simulink library "MEKF_ValidityTest_Lib2018"  (R2018b)
settings: Solver=VariableStepAuto  StartTime=0.0  StopTime=10.0  RelTol=1e-3
values from neighbouring files (symbols this model uses):
  Beta_init = Beta    [MEKF_ScriptandSimulink_Test.m]
  del_t = tspan(2)-tspan(1)    [MEKF_ScriptandSimulink_Test.m]
  P_sq_init = P_sq    [MEKF_ScriptandSimulink_Test.m]
  q = [q(:,2),q(:,3),q(:,4),q(:,1)]    [MEKF_ScriptandSimulink_Test.m]
  Q_sq = chol((gamma*Q_k*gamma'),'lower')    [MEKF_ScriptandSimulink_Test.m]
  qe_init = qe    [MEKF_ScriptandSimulink_Test.m]
  R_sq = chol(R,'lower')    [MEKF_ScriptandSimulink_Test.m]
libraries: MEKF_LibraryR2018b x13, aerolibutil x12, dspmtrx3 x7, sharedutil x6, $bdroot x2
(part 1 of 2)
settings Model: Creator=kylle  LastModifiedBy=kylle
settings DataIOCC: ReturnWorkspaceOutputs=on

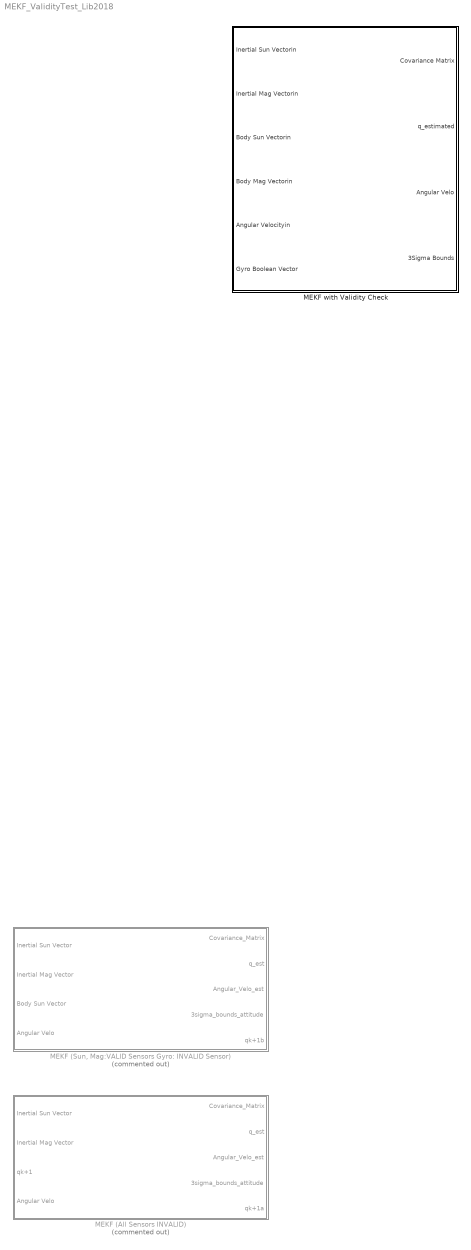
== system MEKF_ValidityTest_Lib2018 ==
  MEKF (All Sensors INVALID) : Subsystem  Commented=on  AncestorBlock=MEKF_Propagation_Lib/MEKF (Gyro Sensors Work, Mag or Sun sensors INVALID)
  "MEKF (Sun, Mag:VALID Sensors Gyro: INVALID Sensor)" : Subsystem  Commented=on  AncestorBlock=MEKF_Propagation_Lib/Multiplicative Extended Kalman Filter (all Valid Sensors)
  MEKF with Validity Check : Subsystem

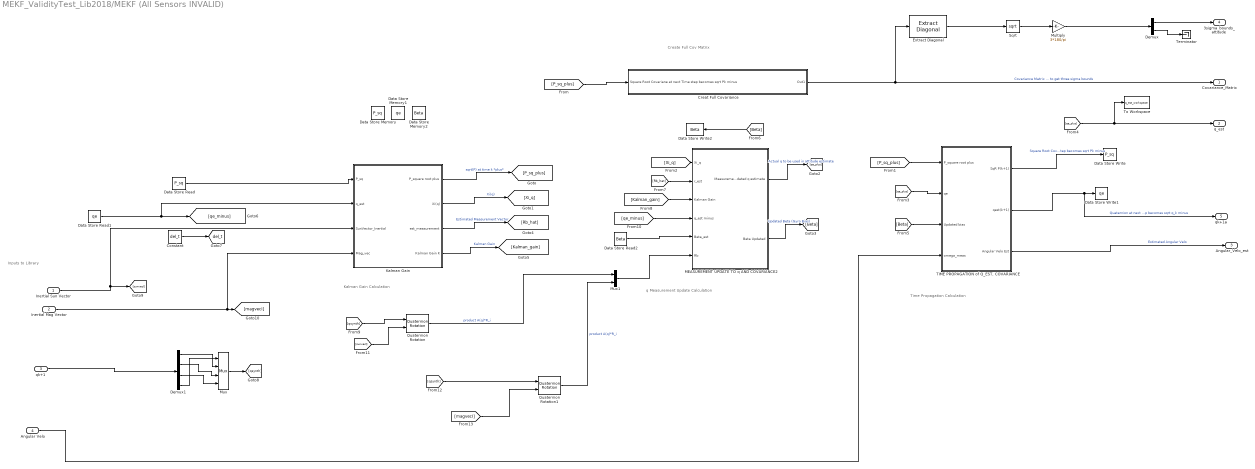
== system MEKF_ValidityTest_Lib2018/MEKF (All Sensors INVALID) ==
  note: Create Full Cov Matrix
  note: Time Propagation Calculation
  note: q Measurement Update Calculation
  note: Inputs to Library
  note: Kalman Gain Calculation
  Inertial Sun Vector : Inport
  Inertial Mag Vector : Inport  Port=2
  qk+1 : Inport  Port=3
  Angular Velo : Inport  Port=4
  Constant : Constant  Value=del_t
  Creat Full Covariance : Subsystem
  Data Store Memory : DataStoreMemory  DataStoreName=P_sq  InitialValue=P_sq_init  VectorParams1D=off  ShowAdditionalParam=off
  Data Store Memory1 : DataStoreMemory  DataStoreName=qe  InitialValue=1000  VectorParams1D=off  ShowAdditionalParam=off
  Data Store Memory2 : DataStoreMemory  DataStoreName=Beta  InitialValue=Beta_init  VectorParams1D=off  ShowAdditionalParam=off
  Data Store Read : DataStoreRead  DataStoreName=P_sq
  Data Store Read1 : DataStoreRead  DataStoreName=qe
  Data Store Read2 : DataStoreRead  DataStoreName=Beta
  Data Store Write : DataStoreWrite  DataStoreName=P_sq
  Data Store Write1 : DataStoreWrite  DataStoreName=qe
  Data Store Write2 : DataStoreWrite  DataStoreName=Beta
  Demux : Demux  Outputs=2
  Demux1 : Demux
  Extract Diagonal : dspmtrx3/Extract Diagonal
      settings: SourceProductName=DSP System Toolbox  SourceProductBaseCode=DS
  Kalman Gain : Subsystem
  MEASUREMENT UPDATE TO q AND COVARIANCE2 : Subsystem
  Multiply : Gain  Gain=3*180/pi
  Mux : Mux
  Mux1 : Mux  Inputs=2
  Quaternion Rotation : aerolibutil/Quaternion Rotation
  Quaternion Rotation1 : aerolibutil/Quaternion Rotation
  Sqrt : Sqrt  SaturateOnIntegerOverflow=on
  "TIME PROPAGATION of Q_EST, COVARIANCE" : Subsystem
  Terminator : Terminator
  To Workspace : ToWorkspace  VariableName=q_est_workspace  SaveFormat=Timeseries  SampleTime=-1
  Covariance_Matrix : Outport
  q_est : Outport  Port=2
  Angular_Velo_est : Outport  Port=3
  3sigma_bounds_attitude : Outport  Port=4
  qk+1a : Outport  Port=5
  tag scope: del_t=global
  wires:
  Data Store Read1/1 -> [qe_minus], Kalman Gain/2(q_est)
  Inertial Mag Vector/1 -> [magvecI], Kalman Gain/4("Mag_vec ")
  Demux/2 -> Terminator/1
  Demux/1 -> 3sigma_bounds_attitude/1
  Multiply/1 -> Demux/1
  Sqrt/1 -> Multiply/1
  Extract Diagonal/1 -> Sqrt/1
  Creat Full Covariance/1(Out1) -> Covariance_Matrix/1, Extract Diagonal/1  "Covariance Matrix from which to get three sigma bounds"
  "TIME PROPAGATION of Q_EST, COVARIANCE"/3(Angular Velo Est) -> Angular_Velo_est/1  "Estimated Angular Velo"
  Angular Velo/1 -> "TIME PROPAGATION of Q_EST, COVARIANCE"/4(omega_meas)
  Kalman Gain/4(Kalman Gain K) -> [Kalman_gain]  "Kalman Gain"
  Inertial Sun Vector/1 -> [sunvecI], Kalman Gain/3(SunVector_Inertial)
  MEASUREMENT UPDATE TO q AND COVARIANCE2/2(Beta Updated) -> [Beta]  "Updated Beta (Gyro Bias)"
  Kalman Gain/3(est_measurement) -> [Rb_hat]  "Estimated Measurement Vector"
  Data Store Read2/1 -> MEASUREMENT UPDATE TO q AND COVARIANCE2/5(Beta_est)
  MEASUREMENT UPDATE TO q AND COVARIANCE2/1(Measurement updated q estimate) -> [qe_plus]  "Actual q to be used in attitude estimate"
  Kalman Gain/1(P_square root plus) -> [P_sq_plus]  "sqrt(P) at time k *plus*"
  [Kalman_gain] -> MEASUREMENT UPDATE TO q AND COVARIANCE2/3(Kalman Gain)
  [qe_minus] -> MEASUREMENT UPDATE TO q AND COVARIANCE2/4(q_est minus)
  [qe_plus] -> "TIME PROPAGATION of Q_EST, COVARIANCE"/2(qe)
  [P_sq_plus] -> "TIME PROPAGATION of Q_EST, COVARIANCE"/1(P_square root plus)
  [Xi_q] -> MEASUREMENT UPDATE TO q AND COVARIANCE2/1(Xi_q)
  Constant/1 -> [del_t]
  "TIME PROPAGATION of Q_EST, COVARIANCE"/1(SqR P(k+1)) -> Data Store Write/1  "Square Root Covariane at next Time step becomes sqrt Pk minus"
  [P_sq_plus] -> Creat Full Covariance/1(Square Root Covariane at next Time step becomes sqrt Pk minus)
  [Beta] -> "TIME PROPAGATION of Q_EST, COVARIANCE"/3(Updated bias)
  [Beta] -> Data Store Write2/1
  Kalman Gain/2(Xi(q)) -> [Xi_q]  "Xi(q)"
  "TIME PROPAGATION of Q_EST, COVARIANCE"/2(qest(k+1)) -> qk+1a/1, Data Store Write1/1  "Quaternion at next Time step becomes sqrt q_k minus"
  Data Store Read/1 -> Kalman Gain/1(P_sq)
  [Rb_hat] -> MEASUREMENT UPDATE TO q AND COVARIANCE2/2(r_est)
  [qe_plus] -> To Workspace/1, q_est/1
  qk+1/1 -> Demux1/1
  Quaternion Rotation/1 -> Mux1/1  "product A(q)*R_i"
  [sunvecI] -> Quaternion Rotation/2
  Demux1/2 -> Mux/3
  Mux/1 -> [qsynth]
  Demux1/3 -> Mux/4
  Demux1/1 -> Mux/2
  Demux1/4 -> Mux/1
  [qsynth] -> Quaternion Rotation/1
  Quaternion Rotation1/1 -> Mux1/2  "product A(q)*R_i"
  [qsynth] -> Quaternion Rotation1/1
  [magvecI] -> Quaternion Rotation1/2
  Mux1/1 -> MEASUREMENT UPDATE TO q AND COVARIANCE2/6(Rb)

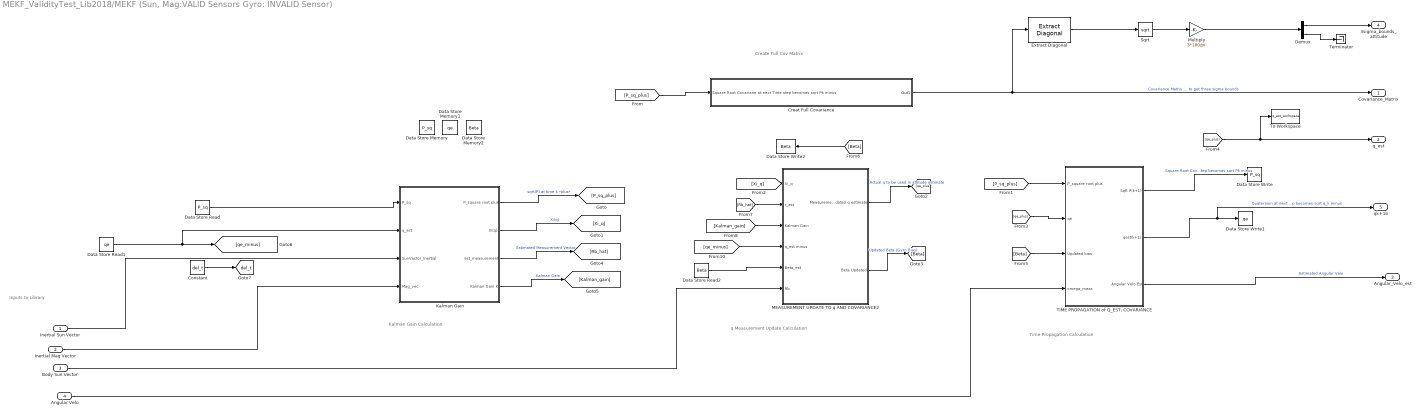
== system MEKF_ValidityTest_Lib2018/MEKF (Sun, Mag:VALID Sensors Gyro: INVALID Sensor) ==
  note: Kalman Gain Calculation
  note: Inputs to Library
  note: q Measurement Update Calculation
  note: Time Propagation Calculation
  note: Create Full Cov Matrix
  Inertial Sun Vector : Inport
  Inertial Mag Vector : Inport  Port=2
  Body Sun Vector : Inport  Port=3
  Angular Velo : Inport  Port=4
  Constant : Constant  Value=del_t
  Creat Full Covariance : Subsystem
  Data Store Memory : DataStoreMemory  DataStoreName=P_sq  InitialValue=P_sq_init  VectorParams1D=off  ShowAdditionalParam=off
  Data Store Memory1 : DataStoreMemory  DataStoreName=qe  InitialValue=1000  VectorParams1D=off  ShowAdditionalParam=off
  Data Store Memory2 : DataStoreMemory  DataStoreName=Beta  InitialValue=Beta_init  VectorParams1D=off  ShowAdditionalParam=off
  Data Store Read : DataStoreRead  DataStoreName=P_sq
  Data Store Read1 : DataStoreRead  DataStoreName=qe
  Data Store Read2 : DataStoreRead  DataStoreName=Beta
  Data Store Write : DataStoreWrite  DataStoreName=P_sq
  Data Store Write1 : DataStoreWrite  DataStoreName=qe
  Data Store Write2 : DataStoreWrite  DataStoreName=Beta
  Demux : Demux  Outputs=2
  Extract Diagonal : dspmtrx3/Extract Diagonal
      settings: SourceProductName=DSP System Toolbox  SourceProductBaseCode=DS
  Kalman Gain : Subsystem
  MEASUREMENT UPDATE TO q AND COVARIANCE2 : Subsystem
  Multiply : Gain  Gain=3*180/pi
  Sqrt : Sqrt  SaturateOnIntegerOverflow=on
  "TIME PROPAGATION of Q_EST, COVARIANCE" : Subsystem
  Terminator : Terminator
  To Workspace : ToWorkspace  VariableName=q_est_workspace  SaveFormat=Timeseries  SampleTime=-1
  Covariance_Matrix : Outport
  q_est : Outport  Port=2
  Angular_Velo_est : Outport  Port=3
  3sigma_bounds_attitude : Outport  Port=4
  qk+1b : Outport  Port=5
  tag scope: del_t=global
  wires:
  [qe_plus] -> q_est/1, To Workspace/1
  [Rb_hat] -> MEASUREMENT UPDATE TO q AND COVARIANCE2/2(r_est)
  Data Store Read/1 -> Kalman Gain/1(P_sq)
  "TIME PROPAGATION of Q_EST, COVARIANCE"/2(qest(k+1)) -> qk+1b/1, Data Store Write1/1  "Quaternion at next Time step becomes sqrt q_k minus"
  Kalman Gain/2(Xi(q)) -> [Xi_q]  "Xi(q)"
  [Beta] -> Data Store Write2/1
  [Beta] -> "TIME PROPAGATION of Q_EST, COVARIANCE"/3(Updated bias)
  [P_sq_plus] -> Creat Full Covariance/1(Square Root Covariane at next Time step becomes sqrt Pk minus)
  "TIME PROPAGATION of Q_EST, COVARIANCE"/1(SqR P(k+1)) -> Data Store Write/1  "Square Root Covariane at next Time step becomes sqrt Pk minus"
  Constant/1 -> [del_t]
  [Xi_q] -> MEASUREMENT UPDATE TO q AND COVARIANCE2/1(Xi_q)
  [P_sq_plus] -> "TIME PROPAGATION of Q_EST, COVARIANCE"/1(P_square root plus)
  [qe_plus] -> "TIME PROPAGATION of Q_EST, COVARIANCE"/2(qe)
  [qe_minus] -> MEASUREMENT UPDATE TO q AND COVARIANCE2/4(q_est minus)
  [Kalman_gain] -> MEASUREMENT UPDATE TO q AND COVARIANCE2/3(Kalman Gain)
  Kalman Gain/1(P_square root plus) -> [P_sq_plus]  "sqrt(P) at time k *plus*"
  MEASUREMENT UPDATE TO q AND COVARIANCE2/1(Measurement updated q estimate) -> [qe_plus]  "Actual q to be used in attitude estimate"
  Data Store Read2/1 -> MEASUREMENT UPDATE TO q AND COVARIANCE2/5(Beta_est)
  Kalman Gain/3(est_measurement) -> [Rb_hat]  "Estimated Measurement Vector"
  MEASUREMENT UPDATE TO q AND COVARIANCE2/2(Beta Updated) -> [Beta]  "Updated Beta (Gyro Bias)"
  Inertial Sun Vector/1 -> Kalman Gain/3(SunVector_Inertial)
  Kalman Gain/4(Kalman Gain K) -> [Kalman_gain]  "Kalman Gain"
  Angular Velo/1 -> "TIME PROPAGATION of Q_EST, COVARIANCE"/4(omega_meas)
  "TIME PROPAGATION of Q_EST, COVARIANCE"/3(Angular Velo Est) -> Angular_Velo_est/1  "Estimated Angular Velo"
  Creat Full Covariance/1(Out1) -> Extract Diagonal/1, Covariance_Matrix/1  "Covariance Matrix from which to get three sigma bounds"
  Extract Diagonal/1 -> Sqrt/1
  Sqrt/1 -> Multiply/1
  Multiply/1 -> Demux/1
  Demux/1 -> 3sigma_bounds_attitude/1
  Demux/2 -> Terminator/1
  Body Sun Vector/1 -> MEASUREMENT UPDATE TO q AND COVARIANCE2/6(Rb)
  Inertial Mag Vector/1 -> Kalman Gain/4("Mag_vec ")
  Data Store Read1/1 -> Kalman Gain/2(q_est), [qe_minus]

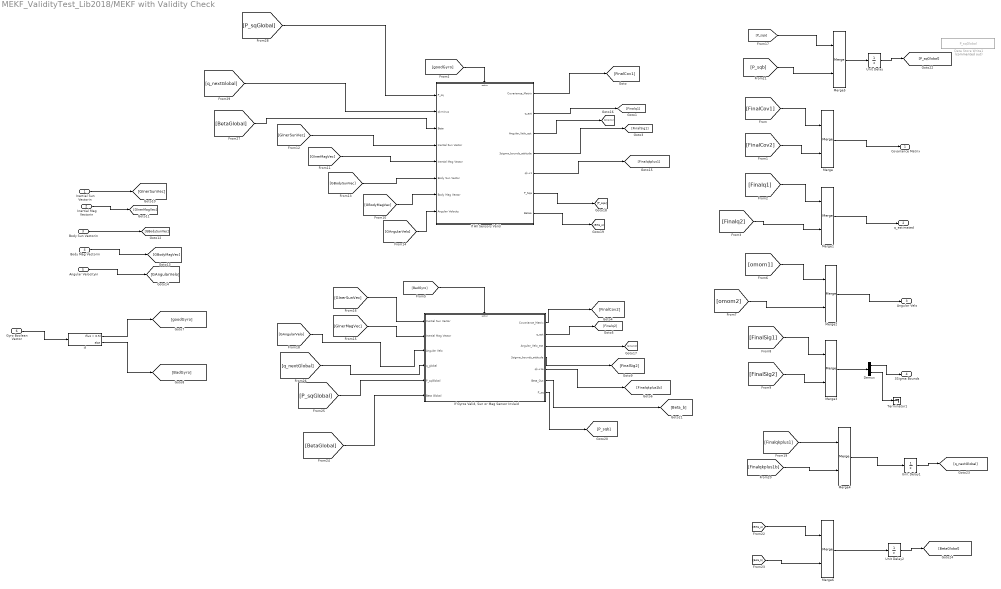
== system MEKF_ValidityTest_Lib2018/MEKF with Validity Check ==
  Inertial Sun Vectorin : Inport
  Inertial Mag Vectorin : Inport  Port=2
  Body Sun Vectorin : Inport  Port=3
  Body Mag Vectorin : Inport  Port=4
  Angular Velocityin : Inport  Port=5
  Gyro Boolean Vector : Inport  Port=6
  Data Store Write1 : DataStoreWrite  Commented=on  DataStoreName=P_sqGlobal
  Demux : Demux  Outputs=2
  If : If  IfExpression=u1 > 0.5
  If All Sensors Valid : Subsystem  TreatAsAtomicUnit=on
  "If Gyros Valid, Sun or Mag Sensor Invlaid" : Subsystem  TreatAsAtomicUnit=on
  Merge{,1..6} (7 alike) : Merge
  Terminator1 : Terminator
  Unit Delay : UnitDelay  InitialCondition=P_sq_init  SampleTime=-1  HasFrameUpgradeWarning=on
  Unit Delay1 : UnitDelay  InitialCondition=qe_init  SampleTime=-1  HasFrameUpgradeWarning=on
  Unit Delay2 : UnitDelay  InitialCondition=Beta_init  SampleTime=-1  HasFrameUpgradeWarning=on
  Covariance Matrix : Outport
  q_estimated : Outport  Port=2
  Angular Velo : Outport  Port=3
  3Sigma Bounds : Outport  Port=4
  wires:
  [GBodySunVec] -> If All Sensors Valid/6(Body Sun Vector)
  [FinalCov2] -> Merge/2
  [GInerMagVec] -> "If Gyros Valid, Sun or Mag Sensor Invlaid"/2(Inertial Mag Vector)
  Gyro Boolean Vector/1 -> If/1
  [GInerMagVec] -> If All Sensors Valid/5(Inertial Mag Vector)
  Body Mag Vectorin/1 -> [GBodyMagVec]
  Merge1/1 -> q_estimated/1
  [GBodyMagVec] -> If All Sensors Valid/7(Body Mag Vector)
  [FinalSig2] -> Merge3/2
  Body Sun Vectorin/1 -> [GBodySunVec]
  [GAngularVelo] -> If All Sensors Valid/8(Angular Velocity)
  "If Gyros Valid, Sun or Mag Sensor Invlaid"/5(qk+1a) -> [Finalqkplus1b]
  If All Sensors Valid/2(q_est) -> [Finalq1]
  If All Sensors Valid/1(Covariance_Matrix) -> [FinalCov1]
  [FinalSig1] -> Merge3/1
  Angular Velocityin/1 -> [GAngularVelo]
  [BadGyro] -> "If Gyros Valid, Sun or Mag Sensor Invlaid"/Action
  [GInerSunVec] -> "If Gyros Valid, Sun or Mag Sensor Invlaid"/1(Inertial Sun Vector)
  [GAngularVelo] -> "If Gyros Valid, Sun or Mag Sensor Invlaid"/3(Angular Velo)
  If All Sensors Valid/4(3sigma_bounds_attitude) -> [FinalSig1]
  Inertial Sun Vectorin/1 -> [GInerSunVec]
  "If Gyros Valid, Sun or Mag Sensor Invlaid"/2(q_est) -> [Finalq2]
  [GInerSunVec] -> If All Sensors Valid/4(Inertial Sun Vector)
  Merge2/1 -> Angular Velo/1
  "If Gyros Valid, Sun or Mag Sensor Invlaid"/1(Covariance_Matrix) -> [FinalCov2]
  [goodGyro] -> If All Sensors Valid/Action
  [Finalq1] -> Merge1/1
  "If Gyros Valid, Sun or Mag Sensor Invlaid"/4(3sigma_bounds_attitude) -> [FinalSig2]
  Merge/1 -> Covariance Matrix/1
  [FinalCov1] -> Merge/1
  [q_nextGlobal] -> "If Gyros Valid, Sun or Mag Sensor Invlaid"/4(q_global)
  Inertial Mag Vectorin/1 -> [GInerMagVec]
  If All Sensors Valid/5(qk+1) -> [Finalqkplus1]
  Merge3/1 -> Demux/1
  Demux/1 -> 3Sigma Bounds/1
  Demux/2 -> Terminator1/1
  [P_sqGlobal] -> "If Gyros Valid, Sun or Mag Sensor Invlaid"/5(P_sqGlobal)
  [Finalqkplus1] -> Merge4/1
  [Finalqkplus1b] -> Merge4/2
  [BetaGlobal] -> "If Gyros Valid, Sun or Mag Sensor Invlaid"/6(Beta Global)
  [BetaGlobal] -> If All Sensors Valid/3(Beta)
  [omom1] -> Merge2/1
  If All Sensors Valid/3(Angular_Velo_est) -> [omom1]
  If All Sensors Valid/6("P_Sqa ") -> [P_sqa]
  If All Sensors Valid/7(Betaa) -> [Beta_a]
  [P_sqa] -> Merge5/1
  "If Gyros Valid, Sun or Mag Sensor Invlaid"/7(P_sq) -> [P_sqb]
  "If Gyros Valid, Sun or Mag Sensor Invlaid"/6(Beta_Out) -> [Beta_b]
  [P_sqb] -> Merge5/2
  "If Gyros Valid, Sun or Mag Sensor Invlaid"/3(Angular_Velo_est) -> [omom2]
  [omom2] -> Merge2/2
  [Beta_a] -> Merge6/1
  [Beta_b] -> Merge6/2
  Merge5/1 -> Unit Delay/1
  Unit Delay/1 -> [P_sqGlobal]
  Unit Delay1/1 -> [q_nextGlobal]
  Merge4/1 -> Unit Delay1/1
  Unit Delay2/1 -> [BetaGlobal]
  Merge6/1 -> Unit Delay2/1
  [q_nextGlobal] -> If All Sensors Valid/2(qkminus)
  [P_sqGlobal] -> If All Sensors Valid/1(P_sq)
  If/1 -> [goodGyro]
  If/2 -> [BadGyro]
  [Finalq2] -> Merge1/2

== system MEKF_ValidityTest_Lib2018/MEKF (All Sensors INVALID)/Creat Full Covariance ==
  Square Root Covariane at next Time step becomes sqrt Pk minus : Inport
  Matrix Multiply : Product  Multiplication=Matrix(*)
  Transpose : Math  Operator=transpose  SaturateOnIntegerOverflow=on
  Out1 : Outport
  wires:
  Matrix Multiply/1 -> Out1/1
  Transpose/1 -> Matrix Multiply/2
  Square Root Covariane at next Time step becomes sqrt Pk minus/1 -> Matrix Multiply/1, Transpose/1

== system MEKF_ValidityTest_Lib2018/MEKF (All Sensors INVALID)/Kalman Gain ==
  P_sq : Inport
  q_est : Inport  Port=2
  SunVector_Inertial : Inport  Port=3
  "Mag_vec " : Inport  Port=4
  Constant : Constant  Value=R_sq*10000  VectorParams1D=off
  Create H matrix : Subsystem
  Demux : Demux
  Divide : Product  Inputs=/  Multiplication=Matrix(*)
  MATLAB Function2 : MATLAB Function  TreatAsAtomicUnit=on
  MATLAB Function3 : MATLAB Function  Commented=on  TreatAsAtomicUnit=on
  MATLAB Function4 : MATLAB Function  Commented=on  TreatAsAtomicUnit=on
  Makes Xi(q) Matrix : Subsystem
  Matrix Concatenate : Concatenate  Mode=Multidimensional array
  Matrix Multiply1 : Product  Multiplication=Matrix(*)
  Mux : Mux
  Quaternion Rotation : aerolibutil/Quaternion Rotation
  Quaternion Rotation1 : aerolibutil/Quaternion Rotation
  P_square root plus : Outport
  Xi(q) : Outport  Port=2
  est_measurement : Outport  Port=3
  Kalman Gain K : Outport  Port=4
  wires:
  Matrix Concatenate/1 -> est_measurement/1
  [bhat] -> Matrix Concatenate/2
  [rb_hat] -> Matrix Concatenate/1
  [bhat] -> Create H matrix/2(bb_hat)
  [qmix] -> Quaternion Rotation/1
  [qmix] -> Quaternion Rotation1/1
  Mux/1 -> [qmix]
  Quaternion Rotation1/1 -> [bhat]  "product A(q)*B_i"
  "Mag_vec "/1 -> Quaternion Rotation1/2
  [rb_hat] -> Create H matrix/1(rb_hat)
  Quaternion Rotation/1 -> [rb_hat]  "product A(q)*R_i"
  [q_est] -> Makes Xi(q) Matrix/1(qest)
  [q_est] -> Demux/1
  q_est/1 -> [q_est]
  Makes Xi(q) Matrix/1(Xi(q)) -> Xi(q)/1
  Demux/4 -> Mux/1
  Demux/3 -> Mux/4
  Demux/2 -> Mux/3
  Demux/1 -> Mux/2
  MATLAB Function2/3(P_sq) -> P_square root plus/1  "P_square root plus"
  Constant/1 -> MATLAB Function2/1(R_sq)
  SunVector_Inertial/1 -> Quaternion Rotation/2
  Matrix Multiply1/1 -> Kalman Gain K/1  "Kalman Gain K"
  P_sq/1 -> MATLAB Function2/2("P_sq ")
  MATLAB Function2/2(sq_Bk) -> Divide/1
  Create H matrix/1(H) -> MATLAB Function2/3(H)  "Sensitivity Matrix"
  MATLAB Function2/1(W) -> Matrix Multiply1/1
  Divide/1 -> Matrix Multiply1/2

== system MEKF_ValidityTest_Lib2018/MEKF (All Sensors INVALID)/MEASUREMENT UPDATE TO q AND COVARIANCE2 ==
  Xi_q : Inport
  r_est : Inport  Port=2
  Kalman Gain : Inport  Port=3
  q_est minus : Inport  Port=4
  Beta_est : Inport  Port=5
  Rb : Inport  Port=6
  Create Measurement Residual : Sum  Inputs=+-
  Demux : Demux  Outputs=2
  Normalize_q : Subsystem
  Product : Product  Inputs=**  Multiplication=Matrix(*)
  Product1 : Product  Multiplication=Matrix(*)
  Sum : Sum  Inputs=|++
  "Updating Beta Bias " : Sum  Inputs=|++
  gain1 : Gain  Gain=0.5
  Measurement updated q estimate : Outport
  Beta Updated : Outport  Port=2
  wires:
  Normalize_q/1(q_normalized) -> Measurement updated q estimate/1
  Sum/1 -> Normalize_q/1(Estimated Quaternion)  "Estimated Quaternion"
  Xi_q/1 -> gain1/1  "quaternion Propagation Matrix"
  Rb/1 -> Create Measurement Residual/1
  Kalman Gain/1 -> Product1/1
  q_est minus/1 -> Sum/2
  Beta_est/1 -> "Updating Beta Bias "/2  "Beta_estimated"
  "Updating Beta Bias "/1 -> Beta Updated/1  "Beta Updated"
  Create Measurement Residual/1 -> Product1/2  "Measurement Residual"
  r_est/1 -> Create Measurement Residual/2
  Product1/1 -> Demux/1  "del_x"
  Product/1 -> Sum/1
  Demux/2 -> "Updating Beta Bias "/1  "Delta Beta"
  gain1/1 -> Product/1  "0.5*Xi_q"
  Demux/1 -> Product/2  "Delta Alpha"

== system MEKF_ValidityTest_Lib2018/MEKF (All Sensors INVALID)/TIME PROPAGATION of Q_EST, COVARIANCE ==
  P_square root plus : Inport
  qe : Inport  Port=2
  Updated bias : Inport  Port=3
  omega_meas : Inport  Port=4
  Constant10 : Constant  Commented=on  Value=del_t
  Constant11 : Constant  Value=0.5
  Constant13 : Constant  Value=Q_sq  VectorParams1D=off
  Goto1 : Goto  Commented=on  GotoTag=del_t
  MATLAB Function : MATLAB Function  TreatAsAtomicUnit=on
  MATLAB Function10 : MATLAB Function  TreatAsAtomicUnit=on
  MATLAB Function11 : MATLAB Function  TreatAsAtomicUnit=on
  MATLAB Function7 : MATLAB Function  TreatAsAtomicUnit=on
  MATLAB Function8 : MATLAB Function  TreatAsAtomicUnit=on
  MATLAB Function9 : MATLAB Function  TreatAsAtomicUnit=on
  Product : Product  Multiplication=Matrix(*)
  Psi : Subsystem
  cos_omega : Subsystem
  subtract bias from omega meas : Sum  Inputs=|-+
  SqR P(k+1) : Outport
  qest(k+1) : Outport  Port=2
  Angular Velo Est : Outport  Port=3
  wires:
  [om_mag] -> Psi/4(In5), Psi/3(In3)
  [omega_est] -> Psi/5(In4)
  Constant11/1 -> Psi/2(In2)
  [del_t] -> Psi/1(In1)
  Psi/1(Psi) -> MATLAB Function7/1(Psi), MATLAB Function8/2(Psi)  "Psi Matrix"
  cos_omega/1(cos_omega) -> MATLAB Function10/2(cos_omega)  "cos_omega"
  [om_mag] -> cos_omega/3(In3)
  [del_t] -> cos_omega/2(In2)
  [om_mag] -> cos_omega/1(In1)
  [qe] -> Product/2
  qe/1 -> [qe]
  [omega_est] -> Angular Velo Est/1
  [omega_est] -> MATLAB Function9/1(omega)
  subtract bias from omega meas/1 -> [omega_est], MATLAB Function/1(omega_est)  "omega est"
  [P_sq_plus] -> MATLAB Function11/3("P_sq ")
  P_square root plus/1 -> [P_sq_plus]
  [del_t] -> MATLAB Function10/1(del_t)
  Constant10/1 -> Goto1/1  "del_t"
  [om_mag] -> MATLAB Function8/3(om_mag)
  [om_mag] -> MATLAB Function10/3(om_mag)
  MATLAB Function/1(om_mag) -> [om_mag]  "om_mag"
  Updated bias/1 -> subtract bias from omega meas/1
  omega_meas/1 -> subtract bias from omega meas/2
  Constant13/1 -> MATLAB Function11/2(Q_sq)  "process noise chol decomped covariance matrix"
  Product/1 -> qest(k+1)/1  "Time Propagated q"
  MATLAB Function10/1(State_Trans_matrix) -> MATLAB Function11/1(Phi_discrete)  "State Transition matrix to proagate P"
  MATLAB Function9/1(omega_cross_matrix) -> MATLAB Function10/4(omega_x)
  MATLAB Function8/1(Omega_omega) -> Product/1  "q propagation matrix (nothing to do with angular velo)"
  MATLAB Function11/1(P_sq) -> SqR P(k+1)/1  "C gets QR decomped to propagate sqrt(P)"
  MATLAB Function7/1(Psi_cross) -> MATLAB Function8/1(Psi_x)
  [del_t] -> MATLAB Function8/4(del_t)

== system MEKF_ValidityTest_Lib2018/MEKF (Sun, Mag:VALID Sensors Gyro: INVALID Sensor)/Creat Full Covariance ==
  Square Root Covariane at next Time step becomes sqrt Pk minus : Inport
  Matrix Multiply : Product  Multiplication=Matrix(*)
  Transpose : Math  Operator=transpose  SaturateOnIntegerOverflow=on
  Out1 : Outport
  wires:
  Square Root Covariane at next Time step becomes sqrt Pk minus/1 -> Transpose/1, Matrix Multiply/1
  Transpose/1 -> Matrix Multiply/2
  Matrix Multiply/1 -> Out1/1

== system MEKF_ValidityTest_Lib2018/MEKF (Sun, Mag:VALID Sensors Gyro: INVALID Sensor)/Kalman Gain ==
  P_sq : Inport
  q_est : Inport  Port=2
  SunVector_Inertial : Inport  Port=3
  "Mag_vec " : Inport  Port=4
  Constant : Constant  Value=R_sq  VectorParams1D=off
  Create H matrix : Subsystem
  Demux : Demux
  Divide : Product  Inputs=/  Multiplication=Matrix(*)
  MATLAB Function2 : MATLAB Function  TreatAsAtomicUnit=on
  MATLAB Function3 : MATLAB Function  Commented=on  TreatAsAtomicUnit=on
  MATLAB Function4 : MATLAB Function  Commented=on  TreatAsAtomicUnit=on
  Makes Xi(q) Matrix : Subsystem
  Matrix Concatenate : Concatenate  Mode=Multidimensional array
  Matrix Multiply1 : Product  Multiplication=Matrix(*)
  Mux : Mux
  Quaternion Rotation : aerolibutil/Quaternion Rotation
  Quaternion Rotation1 : aerolibutil/Quaternion Rotation
  P_square root plus : Outport
  Xi(q) : Outport  Port=2
  est_measurement : Outport  Port=3
  Kalman Gain K : Outport  Port=4
  wires:
  Divide/1 -> Matrix Multiply1/2
  MATLAB Function2/1(W) -> Matrix Multiply1/1
  Create H matrix/1(H) -> MATLAB Function2/3(H)  "Sensitivity Matrix"
  MATLAB Function2/2(sq_Bk) -> Divide/1
  P_sq/1 -> MATLAB Function2/2("P_sq ")
  Matrix Multiply1/1 -> Kalman Gain K/1  "Kalman Gain K"
  SunVector_Inertial/1 -> Quaternion Rotation/2
  Constant/1 -> MATLAB Function2/1(R_sq)
  MATLAB Function2/3(P_sq) -> P_square root plus/1  "P_square root plus"
  Demux/1 -> Mux/2
  Demux/2 -> Mux/3
  Demux/3 -> Mux/4
  Demux/4 -> Mux/1
  Makes Xi(q) Matrix/1(Xi(q)) -> Xi(q)/1
  q_est/1 -> [q_est]
  [q_est] -> Demux/1
  [q_est] -> Makes Xi(q) Matrix/1(qest)
  Quaternion Rotation/1 -> [rb_hat]  "product A(q)*R_i"
  [rb_hat] -> Create H matrix/1(rb_hat)
  "Mag_vec "/1 -> Quaternion Rotation1/2
  Quaternion Rotation1/1 -> [bhat]  "product A(q)*B_i"
  Mux/1 -> [qmix]
  [qmix] -> Quaternion Rotation1/1
  [qmix] -> Quaternion Rotation/1
  [bhat] -> Create H matrix/2(bb_hat)
  [rb_hat] -> Matrix Concatenate/1
  [bhat] -> Matrix Concatenate/2
  Matrix Concatenate/1 -> est_measurement/1

== system MEKF_ValidityTest_Lib2018/MEKF (Sun, Mag:VALID Sensors Gyro: INVALID Sensor)/MEASUREMENT UPDATE TO q AND COVARIANCE2 ==
  Xi_q : Inport
  r_est : Inport  Port=2
  Kalman Gain : Inport  Port=3
  q_est minus : Inport  Port=4
  Beta_est : Inport  Port=5
  Rb : Inport  Port=6
  Create Measurement Residual : Sum  Inputs=+-
  Demux : Demux  Outputs=2
  Normalize_q : Subsystem
  Product : Product  Inputs=**  Multiplication=Matrix(*)
  Product1 : Product  Multiplication=Matrix(*)
  Sum : Sum  Inputs=|++
  "Updating Beta Bias " : Sum  Inputs=|++
  gain1 : Gain  Gain=0.5
  Measurement updated q estimate : Outport
  Beta Updated : Outport  Port=2
  wires:
  Demux/1 -> Product/2  "Delta Alpha"
  gain1/1 -> Product/1  "0.5*Xi_q"
  Demux/2 -> "Updating Beta Bias "/1  "Delta Beta"
  Product/1 -> Sum/1
  Product1/1 -> Demux/1  "del_x"
  r_est/1 -> Create Measurement Residual/2
  Create Measurement Residual/1 -> Product1/2  "Measurement Residual"
  "Updating Beta Bias "/1 -> Beta Updated/1  "Beta Updated"
  Beta_est/1 -> "Updating Beta Bias "/2  "Beta_estimated"
  q_est minus/1 -> Sum/2
  Kalman Gain/1 -> Product1/1
  Rb/1 -> Create Measurement Residual/1
  Xi_q/1 -> gain1/1  "quaternion Propagation Matrix"
  Sum/1 -> Normalize_q/1(Estimated Quaternion)  "Estimated Quaternion"
  Normalize_q/1(q_normalized) -> Measurement updated q estimate/1

== system MEKF_ValidityTest_Lib2018/MEKF (Sun, Mag:VALID Sensors Gyro: INVALID Sensor)/TIME PROPAGATION of Q_EST, COVARIANCE ==
  P_square root plus : Inport
  qe : Inport  Port=2
  Updated bias : Inport  Port=3
  omega_meas : Inport  Port=4
  Constant10 : Constant  Commented=on  Value=del_t
  Constant11 : Constant  Value=0.5
  Constant13 : Constant  Value=Q_sq  VectorParams1D=off
  Goto1 : Goto  Commented=on  GotoTag=del_t
  MATLAB Function : MATLAB Function  TreatAsAtomicUnit=on
  MATLAB Function10 : MATLAB Function  TreatAsAtomicUnit=on
  MATLAB Function11 : MATLAB Function  TreatAsAtomicUnit=on
  MATLAB Function7 : MATLAB Function  TreatAsAtomicUnit=on
  MATLAB Function8 : MATLAB Function  TreatAsAtomicUnit=on
  MATLAB Function9 : MATLAB Function  TreatAsAtomicUnit=on
  Product : Product  Multiplication=Matrix(*)
  Psi : Subsystem
  cos_omega : Subsystem
  subtract bias from omega meas : Sum  Inputs=|-+
  SqR P(k+1) : Outport
  qest(k+1) : Outport  Port=2
  Angular Velo Est : Outport  Port=3
  wires:
  [del_t] -> MATLAB Function8/4(del_t)
  MATLAB Function7/1(Psi_cross) -> MATLAB Function8/1(Psi_x)
  MATLAB Function11/1(P_sq) -> SqR P(k+1)/1  "C gets QR decomped to propagate sqrt(P)"
  MATLAB Function8/1(Omega_omega) -> Product/1  "q propagation matrix (nothing to do with angular velo)"
  MATLAB Function9/1(omega_cross_matrix) -> MATLAB Function10/4(omega_x)
  MATLAB Function10/1(State_Trans_matrix) -> MATLAB Function11/1(Phi_discrete)  "State Transition matrix to proagate P"
  Product/1 -> qest(k+1)/1  "Time Propagated q"
  Constant13/1 -> MATLAB Function11/2(Q_sq)  "process noise chol decomped covariance matrix"
  omega_meas/1 -> subtract bias from omega meas/2
  Updated bias/1 -> subtract bias from omega meas/1
  MATLAB Function/1(om_mag) -> [om_mag]  "om_mag"
  [om_mag] -> MATLAB Function10/3(om_mag)
  [om_mag] -> MATLAB Function8/3(om_mag)
  Constant10/1 -> Goto1/1  "del_t"
  [del_t] -> MATLAB Function10/1(del_t)
  P_square root plus/1 -> [P_sq_plus]
  [P_sq_plus] -> MATLAB Function11/3("P_sq ")
  subtract bias from omega meas/1 -> MATLAB Function/1(omega_est), [omega_est]  "omega est"
  [omega_est] -> MATLAB Function9/1(omega)
  [omega_est] -> Angular Velo Est/1
  qe/1 -> [qe]
  [qe] -> Product/2
  [om_mag] -> cos_omega/1(In1)
  [del_t] -> cos_omega/2(In2)
  [om_mag] -> cos_omega/3(In3)
  cos_omega/1(cos_omega) -> MATLAB Function10/2(cos_omega)  "cos_omega"
  Psi/1(Psi) -> MATLAB Function8/2(Psi), MATLAB Function7/1(Psi)  "Psi Matrix"
  [del_t] -> Psi/1(In1)
  Constant11/1 -> Psi/2(In2)
  [omega_est] -> Psi/5(In4)
  [om_mag] -> Psi/3(In3), Psi/4(In5)

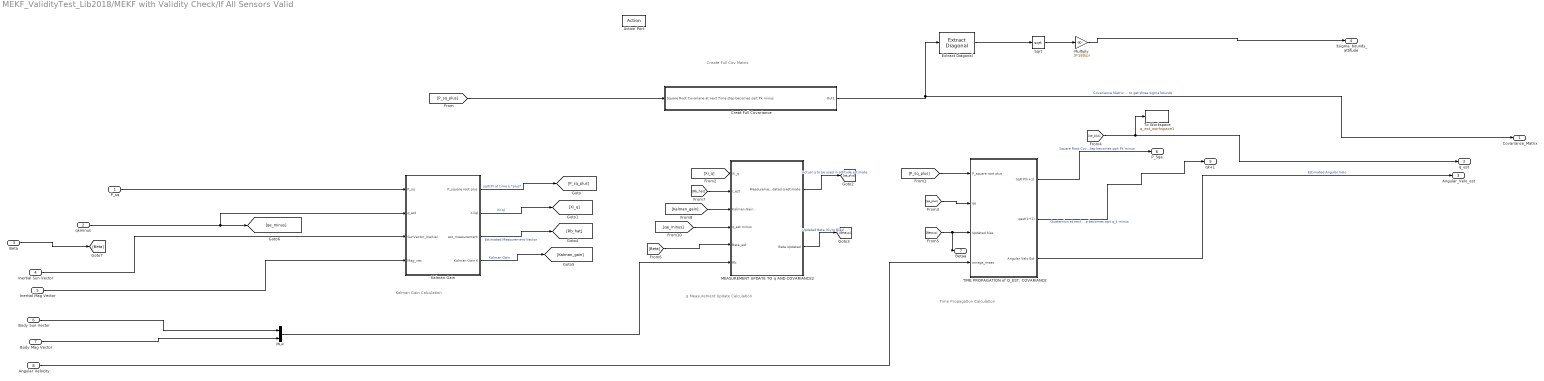
== system MEKF_ValidityTest_Lib2018/MEKF with Validity Check/If All Sensors Valid ==
  note: Kalman Gain Calculation
  note: Time Propagation Calculation
  note: Create Full Cov Matrix
  note: q Measurement Update Calculation
  P_sq : Inport
  qkminus : Inport  Port=2
  Beta : Inport  Port=3
  Inertial Sun Vector : Inport  Port=4
  Inertial Mag Vector : Inport  Port=5
  Body Sun Vector : Inport  Port=6
  Body Mag Vector : Inport  Port=7
  Angular Velocity : Inport  Port=8
  Action Port : ActionPort
  Creat Full Covariance : Subsystem  AncestorBlock=MEKF_LibraryR2018b/Multiplicative Extended Kalman Filter/Creat Full Covariance
  Extract Diagonal : dspmtrx3/Extract Diagonal
      settings: SourceProductName=DSP System Toolbox  SourceProductBaseCode=DS
  Kalman Gain : Subsystem  AncestorBlock=MEKF_LibraryR2018b/Multiplicative Extended Kalman Filter/Kalman Gain
  MEASUREMENT UPDATE TO q AND COVARIANCE2 : Subsystem  AncestorBlock=MEKF_LibraryR2018b/Multiplicative Extended Kalman Filter/MEASUREMENT UPDATE TO q AND COVARIANCE2
  Multiply : Gain  Gain=3*180/pi
  Mux : Mux  Inputs=2
  Sqrt : Sqrt  SaturateOnIntegerOverflow=on
  "TIME PROPAGATION of Q_EST, COVARIANCE" : Subsystem  AncestorBlock=MEKF_Library/Multiplicative Extended Kalman Filter/TIME PROPAGATION of Q_EST, COVARIANCE
  To Workspace : ToWorkspace  VariableName=q_est_workspace1  SaveFormat=Timeseries  SampleTime=-1
  Covariance_Matrix : Outport
  q_est : Outport  Port=2
  Angular_Velo_est : Outport  Port=3
  3sigma_bounds_attitude : Outport  Port=4
  qk+1 : Outport  Port=5
  "P_Sqa " : Outport  Port=6
  Betaa : Outport  Port=7
  wires:
  Inertial Sun Vector/1 -> Kalman Gain/3(SunVector_Inertial)
  [qe_plus] -> q_est/1, To Workspace/1
  "TIME PROPAGATION of Q_EST, COVARIANCE"/2(qest(k+1)) -> qk+1/1  "Quaternion at next Time step becomes sqrt q_k minus"
  "TIME PROPAGATION of Q_EST, COVARIANCE"/3(Angular Velo Est) -> Angular_Velo_est/1  "Estimated Angular Velo"
  Creat Full Covariance/1(Out1) -> Covariance_Matrix/1, Extract Diagonal/1  "Covariance Matrix from which to get three sigma bounds"
  qkminus/1 -> Kalman Gain/2(q_est), [qe_minus]
  Extract Diagonal/1 -> Sqrt/1
  Angular Velocity/1 -> "TIME PROPAGATION of Q_EST, COVARIANCE"/4(omega_meas)
  P_sq/1 -> Kalman Gain/1(P_sq)
  [qe_plus] -> "TIME PROPAGATION of Q_EST, COVARIANCE"/2(qe)
  MEASUREMENT UPDATE TO q AND COVARIANCE2/2(Beta Updated) -> [Betaup]  "Updated Beta (Gyro Bias)"
  [Rb_hat] -> MEASUREMENT UPDATE TO q AND COVARIANCE2/2(r_est)
  "TIME PROPAGATION of Q_EST, COVARIANCE"/1(SqR P(k+1)) -> "P_Sqa "/1  "Square Root Covariane at next Time step becomes sqrt Pk minus"
  Kalman Gain/1(P_square root plus) -> [P_sq_plus]  "sqrt(P) at time k *plus*"
  Kalman Gain/4(Kalman Gain K) -> [Kalman_gain]  "Kalman Gain"
  [qe_minus] -> MEASUREMENT UPDATE TO q AND COVARIANCE2/4(q_est minus)
  Kalman Gain/2(Xi(q)) -> [Xi_q]  "Xi(q)"
  Sqrt/1 -> Multiply/1
  [P_sq_plus] -> Creat Full Covariance/1(Square Root Covariane at next Time step becomes sqrt Pk minus)
  [Betaup] -> Betaa/1, "TIME PROPAGATION of Q_EST, COVARIANCE"/3(Updated bias)
  [Beta] -> MEASUREMENT UPDATE TO q AND COVARIANCE2/5(Beta_est)
  MEASUREMENT UPDATE TO q AND COVARIANCE2/1(Measurement updated q estimate) -> [qe_plus]  "Actual q to be used in attitude estimate"
  [P_sq_plus] -> "TIME PROPAGATION of Q_EST, COVARIANCE"/1(P_square root plus)
  Kalman Gain/3(est_measurement) -> [Rb_hat]  "Estimated Measurement Vector"
  [Xi_q] -> MEASUREMENT UPDATE TO q AND COVARIANCE2/1(Xi_q)
  [Kalman_gain] -> MEASUREMENT UPDATE TO q AND COVARIANCE2/3(Kalman Gain)
  Inertial Mag Vector/1 -> Kalman Gain/4("Mag_vec ")
  Body Sun Vector/1 -> Mux/1
  Body Mag Vector/1 -> Mux/2
  Mux/1 -> MEASUREMENT UPDATE TO q AND COVARIANCE2/6(Rb)
  Multiply/1 -> 3sigma_bounds_attitude/1
  Beta/1 -> [Beta]

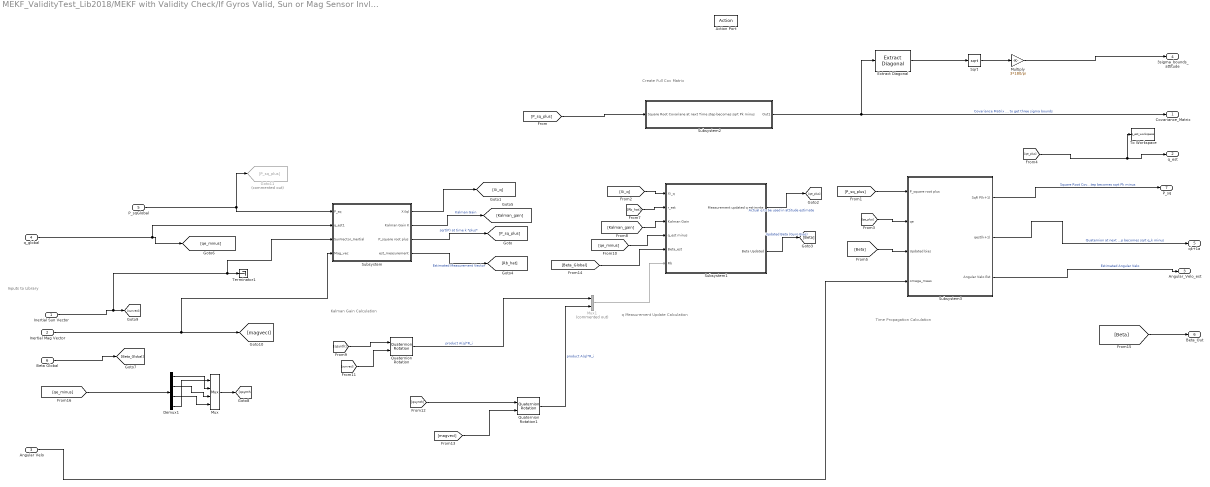
== system MEKF_ValidityTest_Lib2018/MEKF with Validity Check/If Gyros Valid, Sun or Mag Sensor Invlaid ==
  note: q Measurement Update Calculation
  note: Create Full Cov Matrix
  note: Inputs to Library
  note: Kalman Gain Calculation
  note: Time Propagation Calculation
  Inertial Sun Vector : Inport
  Inertial Mag Vector : Inport  Port=2
  Angular Velo : Inport  Port=3
  q_global : Inport  Port=4
  P_sqGlobal : Inport  Port=5
  Beta Global : Inport  Port=6
  Action Port : ActionPort
  Demux1 : Demux
  Extract Diagonal : dspmtrx3/Extract Diagonal
      settings: SourceProductName=DSP System Toolbox  SourceProductBaseCode=DS
  Goto11 : Goto  Commented=on  GotoTag=P_sq_plus
  Multiply : Gain  Gain=3*180/pi
  Mux : Mux
  Mux1 : Mux  Commented=on  Inputs=2
  Quaternion Rotation : aerolibutil/Quaternion Rotation
  Quaternion Rotation1 : aerolibutil/Quaternion Rotation
  Sqrt : Sqrt  SaturateOnIntegerOverflow=on
  Subsystem : Subsystem
  Subsystem1 : Subsystem
  Subsystem2 : Subsystem
  Subsystem3 : Subsystem
  Terminator1 : Terminator
  To Workspace : ToWorkspace  VariableName=q_est_workspace  SaveFormat=Timeseries  SampleTime=-1
  Covariance_Matrix : Outport
  q_est : Outport  Port=2
  Angular_Velo_est : Outport  Port=3
  3sigma_bounds_attitude : Outport  Port=4
  qk+1a : Outport  Port=5
  Beta_Out : Outport  Port=6
  P_sq : Outport  Port=7
  wires:
  Demux1/2 -> Mux/3
  [qsynth] -> Quaternion Rotation/1
  Demux1/1 -> Mux/2
  Demux1/4 -> Mux/1
  Mux/1 -> [qsynth]
  Quaternion Rotation/1 -> Mux1/1  "product A(q)*R_i"
  Quaternion Rotation1/1 -> Mux1/2  "product A(q)*R_i"
  [magvecI] -> Quaternion Rotation1/2
  Demux1/3 -> Mux/4
  Subsystem/4(est_measurement) -> [Rb_hat]  "Estimated Measurement Vector"
  P_sqGlobal/1 -> Subsystem/1(P_sq), Goto11/1
  Subsystem1/1(Measurement updated q estimate) -> [qe_plus]  "Actual q to be used in attitude estimate"
  [qe_plus] -> Subsystem3/2(qe)
  Subsystem3/2(qest(k+1)) -> qk+1a/1  "Quaternion at next Time step becomes sqrt q_k minus"
  Sqrt/1 -> Multiply/1
  Subsystem2/1(Out1) -> Covariance_Matrix/1, Extract Diagonal/1  "Covariance Matrix from which to get three sigma bounds"
  Subsystem/3(P_square root plus) -> [P_sq_plus]  "sqrt(P) at time k *plus*"
  Subsystem1/2(Beta Updated) -> [Beta]  "Updated Beta (Gyro Bias)"
  Subsystem3/3(Angular Velo Est) -> Angular_Velo_est/1  "Estimated Angular Velo"
  [P_sq_plus] -> Subsystem2/1(Square Root Covariane at next Time step becomes sqrt Pk minus)
  [Kalman_gain] -> Subsystem1/3(Kalman Gain)
  [P_sq_plus] -> Subsystem3/1(P_square root plus)
  Subsystem/2(Kalman Gain K) -> [Kalman_gain]  "Kalman Gain"
  [Xi_q] -> Subsystem1/1(Xi_q)
  [Beta] -> Subsystem3/3(Updated bias)
  Extract Diagonal/1 -> Sqrt/1
  q_global/1 -> Subsystem/2(q_est1), [qe_minus]
  Angular Velo/1 -> Subsystem3/4(omega_meas)
  Inertial Mag Vector/1 -> [magvecI], Subsystem/4("Mag_vec ")
  Multiply/1 -> 3sigma_bounds_attitude/1
  Mux1/1 -> Subsystem1/6(Rb)
  Inertial Sun Vector/1 -> Subsystem/3(SunVector_Inertial), Terminator1/1, [sunvecI]
  [Rb_hat] -> Subsystem1/2(r_est)
  [qe_minus] -> Subsystem1/4(q_est minus)
  Subsystem3/1(SqR P(k+1)) -> P_sq/1  "Square Root Covariane at next Time step becomes sqrt Pk minus"
  [qsynth] -> Quaternion Rotation1/1
  [sunvecI] -> Quaternion Rotation/2
  [qe_minus] -> Demux1/1
  Subsystem/1(Xi(q)) -> [Xi_q]
  [Beta_Global] -> Subsystem1/5(Beta_est)
  Beta Global/1 -> [Beta_Global]
  [Beta] -> Beta_Out/1
  [qe_plus] -> To Workspace/1, q_est/1

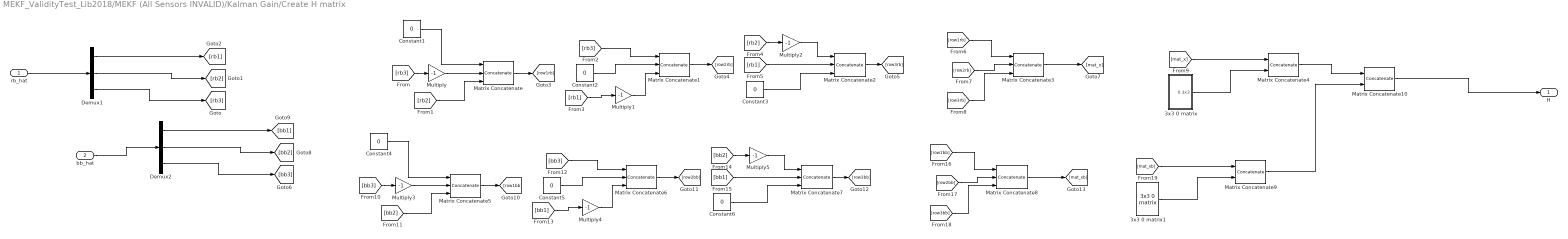
== system MEKF_ValidityTest_Lib2018/MEKF (All Sensors INVALID)/Kalman Gain/Create H matrix ==
  rb_hat : Inport
  bb_hat : Inport  Port=2
  3x3 0 matrix : Subsystem
  3x3 0 matrix1 : $bdroot/Multiplicative Extended Kalman Filter/Kalman Gain/Create H matrix/3x3 0 matrix  SystemSampleTime=-1
  Constant{1..6} (6 alike) : Constant  Value=0
  Demux1 : Demux  Outputs=3
  Demux2 : Demux  Outputs=3
  Matrix Concatenate{,1..2,5..7} (6 alike) : Concatenate  NumInputs=3  Mode=Multidimensional array  ConcatenateDimension=2
  Matrix Concatenate10 : Concatenate  Mode=Multidimensional array
  Matrix Concatenate3 : Concatenate  NumInputs=3  Mode=Multidimensional array
  Matrix Concatenate4 : Concatenate  Mode=Multidimensional array  ConcatenateDimension=2
  Matrix Concatenate8 : Concatenate  NumInputs=3  Mode=Multidimensional array
  Matrix Concatenate9 : Concatenate  Mode=Multidimensional array  ConcatenateDimension=2
  Multiply{,1..5} (6 alike) : Gain  Gain=-1
  H : Outport
  wires:
  Matrix Concatenate10/1 -> H/1
  Matrix Concatenate4/1 -> Matrix Concatenate10/1
  [mat_xb] -> Matrix Concatenate9/1
  Matrix Concatenate9/1 -> Matrix Concatenate10/2
  3x3 0 matrix1/1 -> Matrix Concatenate9/2
  [row3bb] -> Matrix Concatenate8/3
  [row2bb] -> Matrix Concatenate8/2
  Matrix Concatenate8/1 -> [mat_xb]
  [row1bb] -> Matrix Concatenate8/1
  Matrix Concatenate6/1 -> [row2bb]
  [bb2] -> Multiply5/1
  [bb3] -> Matrix Concatenate6/1
  [bb3] -> Multiply3/1
  [bb2] -> Matrix Concatenate5/3
  Constant6/1 -> Matrix Concatenate7/3
  Matrix Concatenate7/1 -> [row3bb]
  [bb1] -> Multiply4/1
  Matrix Concatenate5/1 -> [row1bb]
  Multiply4/1 -> Matrix Concatenate6/3
  Constant5/1 -> Matrix Concatenate6/2
  Multiply3/1 -> Matrix Concatenate5/2
  Constant4/1 -> Matrix Concatenate5/1
  [bb1] -> Matrix Concatenate7/2
  Multiply5/1 -> Matrix Concatenate7/1
  Demux2/2 -> [bb2]
  Demux2/1 -> [bb1]
  bb_hat/1 -> Demux2/1
  Demux2/3 -> [bb3]
  rb_hat/1 -> Demux1/1
  Demux1/3 -> [rb3]
  [rb1] -> Matrix Concatenate2/2
  Constant2/1 -> Matrix Concatenate1/2
  Matrix Concatenate3/1 -> [mat_x]
  Demux1/1 -> [rb1]
  [row1rb] -> Matrix Concatenate3/1
  Constant1/1 -> Matrix Concatenate/1
  [row2rb] -> Matrix Concatenate3/2
  [rb3] -> Matrix Concatenate1/1
  [rb2] -> Matrix Concatenate/3
  [rb2] -> Multiply2/1
  3x3 0 matrix/1(0 3x3) -> Matrix Concatenate4/2
  Constant3/1 -> Matrix Concatenate2/3
  Multiply1/1 -> Matrix Concatenate1/3
  [rb3] -> Multiply/1
  [rb1] -> Multiply1/1
  Matrix Concatenate2/1 -> [row3rb]
  Matrix Concatenate/1 -> [row1rb]
  [row3rb] -> Matrix Concatenate3/3
  Multiply2/1 -> Matrix Concatenate2/1
  Demux1/2 -> [rb2]
  [mat_x] -> Matrix Concatenate4/1
  Multiply/1 -> Matrix Concatenate/2
  Matrix Concatenate1/1 -> [row2rb]

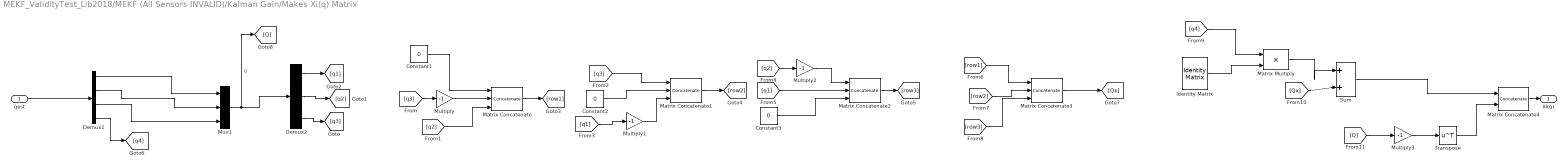
== system MEKF_ValidityTest_Lib2018/MEKF (All Sensors INVALID)/Kalman Gain/Makes Xi(q) Matrix ==
  qest : Inport
  Constant1 : Constant  Value=0
  Constant2 : Constant  Value=0
  Constant3 : Constant  Value=0
  Demux1 : Demux
  Demux2 : Demux  Outputs=3
  Identity Matrix : dspmtrx3/Identity Matrix  Inherit=off  N=3  Ts=1  dataType=double  isSigned=on  wordLen=16  udDataType=sfix(16)  fracBitsMode=Best precision  numFracBits=15  OutDataTypeStr=double  LastOutDataTypeStr=double
      settings: SourceProductName=DSP System Toolbox
  Matrix Concatenate : Concatenate  NumInputs=3  Mode=Multidimensional array  ConcatenateDimension=2
  Matrix Concatenate1 : Concatenate  NumInputs=3  Mode=Multidimensional array  ConcatenateDimension=2
  Matrix Concatenate2 : Concatenate  NumInputs=3  Mode=Multidimensional array  ConcatenateDimension=2
  Matrix Concatenate3 : Concatenate  NumInputs=3  Mode=Multidimensional array
  Matrix Concatenate4 : Concatenate  Mode=Multidimensional array
  Matrix Multiply : Product  Inputs=**
  Multiply{,1..3} (4 alike) : Gain  Gain=-1
  Mux1 : Mux  Inputs=3
  Sum : Sum  Inputs=|++
  Transpose : Math  Operator=transpose  SaturateOnIntegerOverflow=on
  Xi(q) : Outport
  wires:
  Matrix Concatenate4/1 -> Xi(q)/1
  Multiply1/1 -> Matrix Concatenate1/3
  [q1] -> Multiply1/1
  Constant3/1 -> Matrix Concatenate2/3
  Demux2/3 -> [q3]
  Matrix Concatenate/1 -> [row1]
  [q3] -> Multiply/1
  Identity Matrix/1 -> Matrix Multiply/2
  Transpose/1 -> Matrix Concatenate4/2
  Demux2/1 -> [q1]
  [Q] -> Multiply3/1
  [row1] -> Matrix Concatenate3/1
  Multiply/1 -> Matrix Concatenate/2
  [Qx] -> Sum/2
  Matrix Concatenate2/1 -> [row3]
  Demux1/3 -> Mux1/3
  Demux1/1 -> Mux1/1
  [row2] -> Matrix Concatenate3/2
  Demux1/4 -> [q4]
  [q2] -> Multiply2/1
  Sum/1 -> Matrix Concatenate4/1
  Demux2/2 -> [q2]
  [q3] -> Matrix Concatenate1/1
  [q4] -> Matrix Multiply/1
  Multiply3/1 -> Transpose/1
  qest/1 -> Demux1/1
  [row3] -> Matrix Concatenate3/3
  Demux1/2 -> Mux1/2
  Constant2/1 -> Matrix Concatenate1/2
  Mux1/1 -> [Q], Demux2/1  "Q"
  [q2] -> Matrix Concatenate/3
  Matrix Concatenate3/1 -> [Qx]
  Constant1/1 -> Matrix Concatenate/1
  Matrix Concatenate1/1 -> [row2]
  Matrix Multiply/1 -> Sum/1
  [q1] -> Matrix Concatenate2/2
  Multiply2/1 -> Matrix Concatenate2/1

== system MEKF_ValidityTest_Lib2018/MEKF (All Sensors INVALID)/MEASUREMENT UPDATE TO q AND COVARIANCE2/Normalize_q ==
  note: Rearrange_Quat_back
  note: Rearrange_Quat
  Estimated Quaternion : Inport
  Demux : Demux
  Demux1 : Demux
  Mux : Mux
  Mux1 : Mux
  Quaternion Normalize : sharedutil/Quaternion Normalize  aMode=aMode
      settings: SourceProductName=Aerospace Blockset  SourceProductBaseCode=AE
  q_normalized : Outport
  wires:
  Estimated Quaternion/1 -> Demux1/1
  Quaternion Normalize/1 -> Demux/1  "Measurement updated q estimate"
  Demux/1 -> Mux/4
  Demux1/2 -> Mux1/3
  Demux1/1 -> Mux1/2
  Mux/1 -> q_normalized/1
  Demux1/3 -> Mux1/4
  Demux/2 -> Mux/1
  Demux/3 -> Mux/2
  Demux/4 -> Mux/3
  Demux1/4 -> Mux1/1
  Mux1/1 -> Quaternion Normalize/1

== system MEKF_ValidityTest_Lib2018/MEKF (All Sensors INVALID)/TIME PROPAGATION of Q_EST, COVARIANCE/Psi ==
  In1 : Inport
  In2 : Inport  Port=2
  In3 : Inport  Port=3
  In5 : Inport  Port=4
  In4 : Inport  Port=5
  Divide : Product  Inputs=***
  Divide1 : Product  Inputs=**/
  Sin : Trigonometry
  Psi : Outport
  wires:
  In2/1 -> Divide/2
  Sin/1 -> Divide1/1  "sin(om_mag*0.5*del_t)"
  In3/1 -> Divide/3
  Divide1/1 -> Psi/1  "Psi"
  In4/1 -> Divide1/2
  In5/1 -> Divide1/3
  Divide/1 -> Sin/1  "om_mag times0.5*del_t"
  In1/1 -> Divide/1

== system MEKF_ValidityTest_Lib2018/MEKF (All Sensors INVALID)/TIME PROPAGATION of Q_EST, COVARIANCE/cos_omega ==
  In1 : Inport
  In2 : Inport  Port=2
  In3 : Inport  Port=3
  Constant12 : Constant
  Cos : Trigonometry  Operator=cos
  Divide2 : Product  Inputs=**
  Divide3 : Product  Inputs=*/
  Square : Math  Operator=square  SaturateOnIntegerOverflow=on
  Sum3 : Sum  Inputs=|+-
  cos_omega : Outport
  wires:
  Sum3/1 -> Divide3/1  "(1-cos(om_mag*del_t))"
  In2/1 -> Divide2/2
  Cos/1 -> Sum3/2
  In1/1 -> Divide2/1
  Square/1 -> Divide3/2  "omega mag squared"
  Constant12/1 -> Sum3/1
  Divide3/1 -> cos_omega/1  "cos_omega"
  In3/1 -> Square/1
  Divide2/1 -> Cos/1

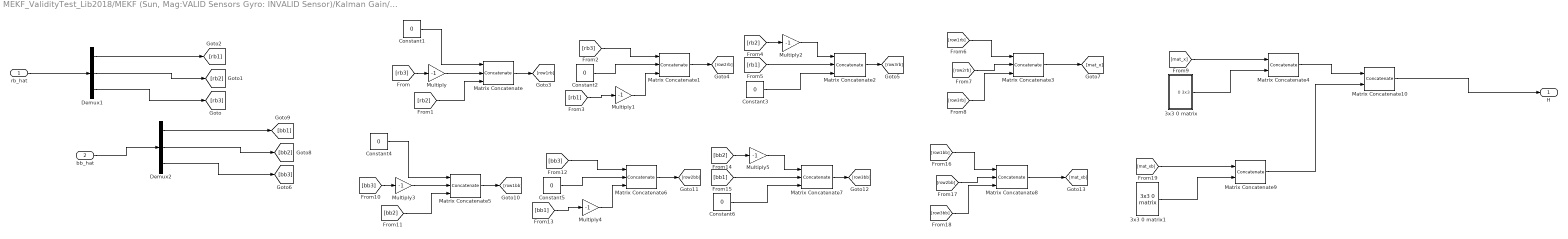
== system MEKF_ValidityTest_Lib2018/MEKF (Sun, Mag:VALID Sensors Gyro: INVALID Sensor)/Kalman Gain/Create H matrix ==
  rb_hat : Inport
  bb_hat : Inport  Port=2
  3x3 0 matrix : Subsystem
  3x3 0 matrix1 : $bdroot/Multiplicative Extended Kalman Filter/Kalman Gain/Create H matrix/3x3 0 matrix  SystemSampleTime=-1
  Constant{1..6} (6 alike) : Constant  Value=0
  Demux1 : Demux  Outputs=3
  Demux2 : Demux  Outputs=3
  Matrix Concatenate{,1..2,5..7} (6 alike) : Concatenate  NumInputs=3  Mode=Multidimensional array  ConcatenateDimension=2
  Matrix Concatenate10 : Concatenate  Mode=Multidimensional array
  Matrix Concatenate3 : Concatenate  NumInputs=3  Mode=Multidimensional array
  Matrix Concatenate4 : Concatenate  Mode=Multidimensional array  ConcatenateDimension=2
  Matrix Concatenate8 : Concatenate  NumInputs=3  Mode=Multidimensional array
  Matrix Concatenate9 : Concatenate  Mode=Multidimensional array  ConcatenateDimension=2
  Multiply{,1..5} (6 alike) : Gain  Gain=-1
  H : Outport
  wires:
  Matrix Concatenate1/1 -> [row2rb]
  Multiply/1 -> Matrix Concatenate/2
  [mat_x] -> Matrix Concatenate4/1
  Demux1/2 -> [rb2]
  Multiply2/1 -> Matrix Concatenate2/1
  [row3rb] -> Matrix Concatenate3/3
  Matrix Concatenate/1 -> [row1rb]
  Matrix Concatenate2/1 -> [row3rb]
  [rb1] -> Multiply1/1
  [rb3] -> Multiply/1
  Multiply1/1 -> Matrix Concatenate1/3
  Constant3/1 -> Matrix Concatenate2/3
  3x3 0 matrix/1(0 3x3) -> Matrix Concatenate4/2
  [rb2] -> Multiply2/1
  [rb2] -> Matrix Concatenate/3
  [rb3] -> Matrix Concatenate1/1
  [row2rb] -> Matrix Concatenate3/2
  Constant1/1 -> Matrix Concatenate/1
  [row1rb] -> Matrix Concatenate3/1
  Demux1/1 -> [rb1]
  Matrix Concatenate3/1 -> [mat_x]
  Constant2/1 -> Matrix Concatenate1/2
  [rb1] -> Matrix Concatenate2/2
  Demux1/3 -> [rb3]
  rb_hat/1 -> Demux1/1
  Demux2/3 -> [bb3]
  bb_hat/1 -> Demux2/1
  Demux2/1 -> [bb1]
  Demux2/2 -> [bb2]
  Multiply5/1 -> Matrix Concatenate7/1
  [bb1] -> Matrix Concatenate7/2
  Constant4/1 -> Matrix Concatenate5/1
  Multiply3/1 -> Matrix Concatenate5/2
  Constant5/1 -> Matrix Concatenate6/2
  Multiply4/1 -> Matrix Concatenate6/3
  Matrix Concatenate5/1 -> [row1bb]
  [bb1] -> Multiply4/1
  Matrix Concatenate7/1 -> [row3bb]
  Constant6/1 -> Matrix Concatenate7/3
  [bb2] -> Matrix Concatenate5/3
  [bb3] -> Multiply3/1
  [bb3] -> Matrix Concatenate6/1
  [bb2] -> Multiply5/1
  Matrix Concatenate6/1 -> [row2bb]
  [row1bb] -> Matrix Concatenate8/1
  Matrix Concatenate8/1 -> [mat_xb]
  [row2bb] -> Matrix Concatenate8/2
  [row3bb] -> Matrix Concatenate8/3
  3x3 0 matrix1/1 -> Matrix Concatenate9/2
  Matrix Concatenate9/1 -> Matrix Concatenate10/2
  [mat_xb] -> Matrix Concatenate9/1
  Matrix Concatenate4/1 -> Matrix Concatenate10/1
  Matrix Concatenate10/1 -> H/1

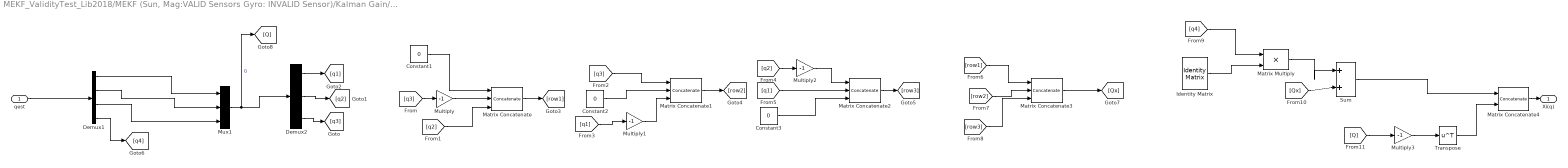
== system MEKF_ValidityTest_Lib2018/MEKF (Sun, Mag:VALID Sensors Gyro: INVALID Sensor)/Kalman Gain/Makes Xi(q) Matrix ==
  qest : Inport
  Constant1 : Constant  Value=0
  Constant2 : Constant  Value=0
  Constant3 : Constant  Value=0
  Demux1 : Demux
  Demux2 : Demux  Outputs=3
  Identity Matrix : dspmtrx3/Identity Matrix  Inherit=off  N=3  Ts=1  dataType=double  isSigned=on  wordLen=16  udDataType=sfix(16)  fracBitsMode=Best precision  numFracBits=15  OutDataTypeStr=double  LastOutDataTypeStr=double
      settings: SourceProductName=DSP System Toolbox
  Matrix Concatenate : Concatenate  NumInputs=3  Mode=Multidimensional array  ConcatenateDimension=2
  Matrix Concatenate1 : Concatenate  NumInputs=3  Mode=Multidimensional array  ConcatenateDimension=2
  Matrix Concatenate2 : Concatenate  NumInputs=3  Mode=Multidimensional array  ConcatenateDimension=2
  Matrix Concatenate3 : Concatenate  NumInputs=3  Mode=Multidimensional array
  Matrix Concatenate4 : Concatenate  Mode=Multidimensional array
  Matrix Multiply : Product  Inputs=**
  Multiply{,1..3} (4 alike) : Gain  Gain=-1
  Mux1 : Mux  Inputs=3
  Sum : Sum  Inputs=|++
  Transpose : Math  Operator=transpose  SaturateOnIntegerOverflow=on
  Xi(q) : Outport
  wires:
  Multiply2/1 -> Matrix Concatenate2/1
  [q1] -> Matrix Concatenate2/2
  Matrix Multiply/1 -> Sum/1
  Matrix Concatenate1/1 -> [row2]
  Constant1/1 -> Matrix Concatenate/1
  Matrix Concatenate3/1 -> [Qx]
  [q2] -> Matrix Concatenate/3
  Mux1/1 -> Demux2/1, [Q]  "Q"
  Constant2/1 -> Matrix Concatenate1/2
  Demux1/2 -> Mux1/2
  [row3] -> Matrix Concatenate3/3
  qest/1 -> Demux1/1
  Multiply3/1 -> Transpose/1
  [q4] -> Matrix Multiply/1
  [q3] -> Matrix Concatenate1/1
  Demux2/2 -> [q2]
  Sum/1 -> Matrix Concatenate4/1
  [q2] -> Multiply2/1
  Demux1/4 -> [q4]
  [row2] -> Matrix Concatenate3/2
  Demux1/1 -> Mux1/1
  Demux1/3 -> Mux1/3
  Matrix Concatenate2/1 -> [row3]
  [Qx] -> Sum/2
  Multiply/1 -> Matrix Concatenate/2
  [row1] -> Matrix Concatenate3/1
  [Q] -> Multiply3/1
  Demux2/1 -> [q1]
  Transpose/1 -> Matrix Concatenate4/2
  Identity Matrix/1 -> Matrix Multiply/2
  [q3] -> Multiply/1
  Matrix Concatenate/1 -> [row1]
  Demux2/3 -> [q3]
  Constant3/1 -> Matrix Concatenate2/3
  [q1] -> Multiply1/1
  Multiply1/1 -> Matrix Concatenate1/3
  Matrix Concatenate4/1 -> Xi(q)/1

== system MEKF_ValidityTest_Lib2018/MEKF (Sun, Mag:VALID Sensors Gyro: INVALID Sensor)/MEASUREMENT UPDATE TO q AND COVARIANCE2/Normalize_q ==
  note: Rearrange_Quat
  note: Rearrange_Quat_back
  Estimated Quaternion : Inport
  Demux : Demux
  Demux1 : Demux
  Mux : Mux
  Mux1 : Mux
  Quaternion Normalize : sharedutil/Quaternion Normalize  aMode=aMode
      settings: SourceProductName=Aerospace Blockset  SourceProductBaseCode=AE
  q_normalized : Outport
  wires:
  Mux1/1 -> Quaternion Normalize/1
  Demux1/4 -> Mux1/1
  Demux/4 -> Mux/3
  Demux/3 -> Mux/2
  Demux/2 -> Mux/1
  Demux1/3 -> Mux1/4
  Mux/1 -> q_normalized/1
  Demux1/1 -> Mux1/2
  Demux1/2 -> Mux1/3
  Demux/1 -> Mux/4
  Quaternion Normalize/1 -> Demux/1  "Measurement updated q estimate"
  Estimated Quaternion/1 -> Demux1/1

== system MEKF_ValidityTest_Lib2018/MEKF (Sun, Mag:VALID Sensors Gyro: INVALID Sensor)/TIME PROPAGATION of Q_EST, COVARIANCE/Psi ==
  In1 : Inport
  In2 : Inport  Port=2
  In3 : Inport  Port=3
  In5 : Inport  Port=4
  In4 : Inport  Port=5
  Divide : Product  Inputs=***
  Divide1 : Product  Inputs=**/
  Sin : Trigonometry
  Psi : Outport
  wires:
  In1/1 -> Divide/1
  Divide/1 -> Sin/1  "om_mag times0.5*del_t"
  In5/1 -> Divide1/3
  In4/1 -> Divide1/2
  Divide1/1 -> Psi/1  "Psi"
  In3/1 -> Divide/3
  Sin/1 -> Divide1/1  "sin(om_mag*0.5*del_t)"
  In2/1 -> Divide/2

== system MEKF_ValidityTest_Lib2018/MEKF (Sun, Mag:VALID Sensors Gyro: INVALID Sensor)/TIME PROPAGATION of Q_EST, COVARIANCE/cos_omega ==
  In1 : Inport
  In2 : Inport  Port=2
  In3 : Inport  Port=3
  Constant12 : Constant
  Cos : Trigonometry  Operator=cos
  Divide2 : Product  Inputs=**
  Divide3 : Product  Inputs=*/
  Square : Math  Operator=square  SaturateOnIntegerOverflow=on
  Sum3 : Sum  Inputs=|+-
  cos_omega : Outport
  wires:
  Divide2/1 -> Cos/1
  In3/1 -> Square/1
  Divide3/1 -> cos_omega/1  "cos_omega"
  Constant12/1 -> Sum3/1
  Square/1 -> Divide3/2  "omega mag squared"
  In1/1 -> Divide2/1
  Cos/1 -> Sum3/2
  In2/1 -> Divide2/2
  Sum3/1 -> Divide3/1  "(1-cos(om_mag*del_t))"

== system MEKF_ValidityTest_Lib2018/MEKF with Validity Check/If All Sensors Valid/Creat Full Covariance ==
  Square Root Covariane at next Time step becomes sqrt Pk minus : Inport
  Matrix Multiply : Product  Multiplication=Matrix(*)
  Transpose : Math  Operator=transpose  SaturateOnIntegerOverflow=on
  Out1 : Outport
  wires:
  Square Root Covariane at next Time step becomes sqrt Pk minus/1 -> Transpose/1, Matrix Multiply/1
  Transpose/1 -> Matrix Multiply/2
  Matrix Multiply/1 -> Out1/1
